simulink model "MAIN_IC_TEST_original"  (R2020b)
settings: Solver=ode4  StartTime=0.0  StopTime=inf  FixedStep=1/1000  RelTol=1e-3
libraries: speedgoatlib_IO691 x12, canmsglib x10, simulink x2
(part 2 of 2)

== matlab function MAIN_IC_TEST_original/to_dPolar1 ==
  data: theta1 input; theta2 input; dr output; dphi output; dtheta1 input; dtheta2 input
function [dr,dphi] = Velocity(theta1,theta2,dtheta1,dtheta2)
%VELOCITY
%    [DR,DPHI] = VELOCITY(THETA1,THETA2,DTHETA1,DTHETA2)

%    This function was generated by the Symbolic Math Toolbox version 8.6.
%    13-May-2022 14:39:46

dr = dtheta1.*1.0./sqrt((sin(acos(sqrt((sin(theta1-pi./2.0).*(3.7e+1./2.0e+2)+sin(theta2+pi./2.0).*(3.7e+1./2.0e+2)).^2+abs(cos(theta1-pi./2.0).*(3.7e+1./2.0e+2)+cos(theta2+pi./2.0).*(3.7e+1./2.0e+2)+3.0./2.5e+1).^2).*(5.0e+1./3.7e+1))+atan2(sin(theta1-pi./2.0).*(-3.7e+1./2.0e+2)-sin(theta2+pi./2.0).*(3.7e+1./2.0e+2),abs(cos(theta1-pi./2.0).*(3.7e+1./2.0e+2)+cos(theta2+pi./2.0).*(3.7e+1./2.0e+2)+3.0./2.5e+1))+7.170057008954915e-2).*4.187654330625071e-1+sin(theta2+pi./2.0).*(3.7e+1./2.0e+2)).^2+(cos(acos(sqrt((sin(theta1-pi./2.0).*(3.7e+1./2.0e+2)+sin(theta2+pi./2.0).*(3.7e+1./2.0e+2)).^2+abs(cos(theta1-pi./2.0).*(3.7e+1./2.0e+2)+cos(theta2+pi./2.0).*(3.7e+1./2.0e+2)+3.0./2.5e+1).^2).*(5.0e+1./3.7e+1))+atan2(sin(theta1-pi./2.0).*(-3.7e+1./2.0e+2)-sin(theta2+pi./2.0).*(3.7e+1./2.0e+2),abs(cos(theta1-pi./2.0).*(3.7e+1./2.0e+2)+cos(theta2+pi./2.0).*(3.7e+1./2.0e+2)+3.0./2.5e+1))+7.170057008954915e-2).*(-4.187654330625071e-1)+cos(theta2+pi./2.0).*(3.7e+1./2.0e+2)+3.0./5.0e+1).^2).*(sin(acos(sqrt((sin(theta1-pi./2.0).*(3.7e+1./2.0e+2)+sin(theta2+pi./2.0).*(3.7e+1./2.0e+2)).^2+abs(cos(theta1-pi./2.0).*(3.7e+1./2.0e+2)+cos(theta2+pi./2.0).*(3.7e+1./2.0e+2)+3.0./2.5e+1).^2).*(5.0e+1./3.7e+1))+atan2(sin(theta1-pi./2.0).*(-3.7e+1./2.0e+2)-sin(theta2+pi./2.0).*(3.7e+1./2.0e+2),abs(cos(theta1-pi./2.0).*(3.7e+1./2.0e+2)+cos(theta2+pi./2.0).*(3.7e+1./2.0e+2)+3.0./2.5e+1))+7.170057008954915e-2).*(1.0./sqrt((sin(theta1-pi./2.0).*(3.7e+1./2.0e+2)+sin(theta2+pi./2.0).*(3.7e+1./2.0e+2)).^2+abs(cos(theta1-pi./2.0).*(3.7e+1./2.0e+2)+cos(theta2+pi./2.0).*(3.7e+1./2.0e+2)+3.0./2.5e+1).^2).*(cos(theta1-pi./2.0).*(sin(theta1-pi./2.0).*(3.7e+1./2.0e+2)+sin(theta2+pi./2.0).*(3.7e+1./2.0e+2)).*(3.7e+1./1.0e+2)-abs(cos(theta1-pi./2.0).*(3.7e+1./2.0e+2)+cos(theta2+pi./2.0).*(3.7e+1./2.0e+2)+3.0./2.5e+1).*sign(cos(theta1-pi./2.0).*(3.7e+1./2.0e+2)+cos(theta2+pi./2.0).*(3.7e+1./2.0e+2)+3.0./2.5e+1).*sin(theta1-pi./2.0).*(3.7e+1./1.0e+2)).*1.0./sqrt((sin(theta1-pi./2.0).*(3.7e+1./2.0e+2)+sin(theta2+pi./2.0).*(3.7e+1./2.0e+2)).^2.*(-1.826150474799123)-abs(cos(theta1-pi./2.0).*(3.7e+1./2.0e+2)+cos(theta2+pi./2.0).*(3.7e+1./2.0e+2)+3.0./2.5e+1).^2.*1.826150474799123+1.0).*(2.5e+1./3.7e+1)+(abs(cos(theta1-pi./2.0).*(3.7e+1./2.0e+2)+cos(theta2+pi./2.0).*(3.7e+1./2.0e+2)+3.0./2.5e+1).^2.*((cos(theta1-pi./2.0).*(3.7e+1./2.0e+2))./abs(cos(theta1-pi./2.0).*(3.7e+1./2.0e+2)+cos(theta2+pi./2.0).*(3.7e+1./2.0e+2)+3.0./2.5e+1)+1.0./abs(cos(theta1-pi./2.0).*(3.7e+1./2.0e+2)+cos(theta2+pi./2.0).*(3.7e+1./2.0e+2)+3.0./2.5e+1).^2.*sign(cos(theta1-pi./2.0).*(3.7e+1./2.0e+2)+cos(theta2+pi./2.0).*(3.7e+1./2.0e+2)+3.0./2.5e+1).*sin(theta1-pi./2.0).*(sin(theta1-pi./2.0).*(3.7e+1./2.0e+2)+sin(theta2+pi./2.0).*(3.7e+1./2.0e+2)).*(3.7e+1./2.0e+2)))./((sin(theta1-pi./2.0).*(3.7e+1./2.0e+2)+sin(theta2+pi./2.0).*(3.7e+1./2.0e+2)).^2+abs(cos(theta1-pi./2.0).*(3.7e+1./2.0e+2)+cos(theta2+pi./2.0).*(3.7e+1./2.0e+2)+3.0./2.5e+1).^2)).*(cos(acos(sqrt((sin(theta1-pi./2.0).*(3.7e+1./2.0e+2)+sin(theta2+pi./2.0).*(3.7e+1./2.0e+2)).^2+abs(cos(theta1-pi./2.0).*(3.7e+1./2.0e+2)+cos(theta2+pi./2.0).*(3.7e+1./2.0e+2)+3.0./2.5e+1).^2).*(5.0e+1./3.7e+1))+atan2(sin(theta1-pi./2.0).*(-3.7e+1./2.0e+2)-sin(theta2+pi./2.0).*(3.7e+1./2.0e+2),abs(cos(theta1-pi./2.0).*(3.7e+1./2.0e+2)+cos(theta2+pi./2.0).*(3.7e+1./2.0e+2)+3.0./2.5e+1))+7.170057008954915e-2).*(-4.187654330625071e-1)+cos(theta2+pi./2.0).*(3.7e+1./2.0e+2)+3.0./5.0e+1).*8.375308661250142e-1+cos(acos(sqrt((sin(theta1-pi./2.0).*(3.7e+1./2.0e+2)+sin(theta2+pi./2.0).*(3.7e+1./2.0e+2)).^2+abs(cos(theta1-pi./2.0).*(3.7e+1./2.0e+2)+cos(theta2+pi./2.0).*(3.7e+1./2.0e+2)+3.0./2.5e+1).^2).*(5.0e+1./3.7e+1))+atan2(sin(theta1-pi./2.0).*(-3.7e+1./2.0e+2)-sin(theta2+pi./2.0).*(3.7e+1./2.0e+2),abs(cos(theta1-pi./2.0).*(3.7e+1./2.0e+2)+cos(theta2+pi./2.0).*(3.7e+1./2.0e+2)+3.0./2.5e+1))+7.170057008954915e-2).*(1.0./sqrt((sin(theta1-pi./2.0).*(3.7e+1./2.0e+2)+sin(theta2+pi./2.0).*(3.7e+1./2.0e+2)).^2+abs(cos(theta1-pi./2.0).*(3.7e+1./2.0e+2)+cos(theta2+pi./2.0).*(3.7e+1./2.0e+2)+3.0./2.5e+1).^2).*(cos(theta1-pi./2.0).*(sin(theta1-pi./2.0).*(3.7e+1./2.0e+2)+sin(theta2+pi./2.0).*(3.7e+1./2.0e+2)).*(3.7e+1./1.0e+2)-abs(cos(theta1-pi./2.0).*(3.7e+1./2.0e+2)+cos(theta2+pi./2.0).*(3.7e+1./2.0e+2)+3.0./2.5e+1).*sign(cos(theta1-pi./2.0).*(3.7e+1./2.0e+2)+cos(theta2+pi./2.0).*(3.7e+1./2.0e+2)+3.0./2.5e+1).*sin(theta1-pi./2.0).*(3.7e+1./1.0e+2)).*1.0./sqrt((sin(theta1-pi./2.0).*(3.7e+1./2.0e+2)+sin(theta2+pi./2.0).*(3.7e+1./2.0e+2)).^2.*(-1.826150474799123)-abs(cos(theta1-pi./2.0).*(3.7e+1./2.0e+2)+cos(theta2+pi./2.0).*(3.7e+1./2.0e+2)+3.0./2.5e+1).^2.*1.826150474799123+1.0).*(2.5e+1./3.7e+1)+(abs(cos(theta1-pi./2.0).*(3.7e+1./2.0e+2)+cos(theta2+pi./2.0).*(3.7e+1./2.0e+2)+3.0./2.5e+1).^2.*((cos(theta1-pi./2.0).*(3.7e+1./2.0e+2))./abs(cos(theta1-pi./2.0).*(3.7e+1./2.0e+2)+cos(theta2+pi./2.0).*(3.7e+1./2.0e+2)+3.0./2.5e+1)+1.0./abs(cos(theta1-pi./2.0).*(3.7e+1./2.0e+2)+cos(theta2+pi./2.0).*(3.7e+1./2.0e+2)+3.0./2.5e+1).^2.*sign(cos(theta1-pi./2.0).*(3.7e+1./2.0e+2)+cos(theta2+pi./2.0).*(3.7e+1./2.0e+2)+3.0./2.5e+1).*sin(theta1-pi./2.0).*(sin(theta1-pi./2.0).*(3.7e+1./2.0e+2)+sin(theta2+pi./2.0).*(3.7e+1./2.0e+2)).*(3.7e+1./2.0e+2)))./((sin(theta1-pi./2.0).*(3.7e+1./2.0e+2)+sin(theta2+pi./2.0).*(3.7e+1./2.0e+2)).^2+abs(cos(theta1-pi./2.0).*(3.7e+1./2.0e+2)+cos(theta2+pi./2.0).*(3.7e+1./2.0e+2)+3.0./2.5e+1).^2)).*(sin(acos(sqrt((sin(theta1-pi./2.0).*(3.7e+1./2.0e+2)+sin(theta2+pi./2.0).*(3.7e+1./2.0e+2)).^2+abs(cos(theta1-pi./2.0).*(3.7e+1./2.0e+2)+cos(theta2+pi./2.0).*(3.7e+1./2.0e+2)+3.0./2.5e+1).^2).*(5.0e+1./3.7e+1))+atan2(sin(theta1-pi./2.0).*(-3.7e+1./2.0e+2)-sin(theta2+pi./2.0).*(3.7e+1./2.0e+2),abs(cos(theta1-pi./2.0).*(3.7e+1./2.0e+2)+cos(theta2+pi./2.0).*(3.7e+1./2.0e+2)+3.0./2.5e+1))+7.170057008954915e-2).*4.187654330625071e-1+sin(theta2+pi./2.0).*(3.7e+1./2.0e+2)).*8.375308661250142e-1).*(-1.0./2.0)+(dtheta2.*1.0./sqrt((sin(acos(sqrt((sin(theta1-pi./2.0).*(3.7e+1./2.0e+2)+sin(theta2+pi./2.0).*(3.7e+1./2.0e+2)).^2+abs(cos(theta1-pi./2.0).*(3.7e+1./2.0e+2)+cos(theta2+pi./2.0).*(3.7e+1./2.0e+2)+3.0./2.5e+1).^2).*(5.0e+1./3.7e+1))+atan2(sin(theta1-pi./2.0).*(-3.7e+1./2.0e+2)-sin(theta2+pi./2.0).*(3.7e+1./2.0e+2),abs(cos(theta1-pi./2.0).*(3.7e+1./2.0e+2)+cos(theta2+pi./2.0).*(3.7e+1./2.0e+2)+3.0./2.5e+1))+7.170057008954915e-2).*4.187654330625071e-1+sin(theta2+pi./2.0).*(3.7e+1./2.0e+2)).^2+(cos(acos(sqrt((sin(theta1-pi./2.0).*(3.7e+1./2.0e+2)+sin(theta2+pi./2.0).*(3.7e+1./2.0e+2)).^2+abs(cos(theta1-pi./2.0).*(3.7e+1./2.0e+2)+cos(theta2+pi./2.0).*(3.7e+1./2.0e+2)+3.0./2.5e+1).^2).*(5.0e+1./3.7e+1))+atan2(sin(theta1-pi./2.0).*(-3.7e+1./2.0e+2)-sin(theta2+pi./2.0).*(3.7e+1./2.0e+2),abs(cos(theta1-pi./2.0).*(3.7e+1./2.0e+2)+cos(theta2+pi./2.0).*(3.7e+1./2.0e+2)+3.0./2.5e+1))+7.170057008954915e-2).*(-4.187654330625071e-1)+cos(theta2+pi./2.0).*(3.7e+1./2.0e+2)+3.0./5.0e+1).^2).*((cos(theta2+pi./2.0).*(3.7e+1./2.0e+2)-cos(acos(sqrt((sin(theta1-pi./2.0).*(3.7e+1./2.0e+2)+sin(theta2+pi./2.0).*(3.7e+1./2.0e+2)).^2+abs(cos(theta1-pi./2.0).*(3.7e+1./2.0e+2)+cos(theta2+pi./2.0).*(3.7e+1./2.0e+2)+3.0./2.5e+1).^2).*(5.0e+1./3.7e+1))+atan2(sin(theta1-pi./2.0).*(-3.7e+1./2.0e+2)-sin(theta2+pi./2.0).*(3.7e+1./2.0e+2),abs(cos(theta1-pi./2.0).*(3.7e+1./2.0e+2)+cos(theta2+pi./2.0).*(3.7e+1./2.0e+2)+3.0./2.5e+1))+7.170057008954915e-2).*(1.0./sqrt((sin(theta1-pi./2.0).*(3.7e+1./2.0e+2)+sin(theta2+pi./2.0).*(3.7e+1./2.0e+2)).^2+abs(cos(theta1-pi./2.0).*(3.7e+1./2.0e+2)+cos(theta2+pi./2.0).*(3.7e+1./2.0e+2)+3.0./2.5e+1).^2).*(cos(theta2+pi./2.0).*(sin(theta1-pi./2.0).*(3.7e+1./2.0e+2)+sin(theta2+pi./2.0).*(3.7e+1./2.0e+2)).*(3.7e+1./1.0e+2)-abs(cos(theta1-pi./2.0).*(3.7e+1./2.0e+2)+cos(theta2+pi./2.0).*(3.7e+1./2.0e+2)+3.0./2.5e+1).*sign(cos(theta1-pi./2.0).*(3.7e+1./2.0e+2)+cos(theta2+pi./2.0).*(3.7e+1./2.0e+2)+3.0./2.5e+1).*sin(theta2+pi./2.0).*(3.7e+1./1.0e+2)).*1.0./sqrt((sin(theta1-pi./2.0).*(3.7e+1./2.0e+2)+sin(theta2+pi./2.0).*(3.7e+1./2.0e+2)).^2.*(-1.826150474799123)-abs(cos(theta1-pi./2.0).*(3.7e+1./2.0e+2)+cos(theta2+pi./2.0).*(3.7e+1./2.0e+2)+3.0./2.5e+1).^2.*1.826150474799123+1.0).*(2.5e+1./3.7e+1)+(abs(cos(theta1-pi./2.0).*(3.7e+1./2.0e+2)+cos(theta2+pi./2.0).*(3.7e+1./2.0e+2)+3.0./2.5e+1).^2.*((cos(theta2+pi./2.0).*(3.7e+1./2.0e+2))./abs(cos(theta1-pi./2.0).*(3.7e+1./2.0e+2)+cos(theta2+pi./2.0).*(3.7e+1./2.0e+2)+3.0./2.5e+1)+1.0./abs(cos(theta1-pi./2.0).*(3.7e+1./2.0e+2)+cos(theta2+pi./2.0).*(3.7e+1./2.0e+2)+3.0./2.5e+1).^2.*sign(cos(theta1-pi./2.0).*(3.7e+1./2.0e+2)+cos(theta2+pi./2.0).*(3.7e+1./2.0e+2)+3.0./2.5e+1).*sin(theta2+pi./2.0).*(sin(theta1-pi./2.0).*(3.7e+1./2.0e+2)+sin(theta2+pi./2.0).*(3.7e+1./2.0e+2)).*(3.7e+1./2.0e+2)))./((sin(theta1-pi./2.0).*(3.7e+1./2.0e+2)+sin(theta2+pi./2.0).*(3.7e+1./2.0e+2)).^2+abs(cos(theta1-pi./2.0).*(3.7e+1./2.0e+2)+cos(theta2+pi./2.0).*(3.7e+1./2.0e+2)+3.0./2.5e+1).^2)).*4.187654330625071e-1).*(sin(acos(sqrt((sin(theta1-pi./2.0).*(3.7e+1./2.0e+2)+sin(theta2+pi./2.0).*(3.7e+1./2.0e+2)).^2+abs(cos(theta1-pi./2.0).*(3.7e+1./2.0e+2)+cos(theta2+pi./2.0).*(3.7e+1./2.0e+2)+3.0./2.5e+1).^2).*(5.0e+1./3.7e+1))+atan2(sin(theta1-pi./2.0).*(-3.7e+1./2.0e+2)-sin(theta2+pi./2.0).*(3.7e+1./2.0e+2),abs(cos(theta1-pi./2.0).*(3.7e+1./2.0e+2)+cos(theta2+pi./2.0).*(3.7e+1./2.0e+2)+3.0./2.5e+1))+7.170057008954915e-2).*4.187654330625071e-1+sin(theta2+pi./2.0).*(3.7e+1./2.0e+2)).*2.0-(sin(theta2+pi./2.0).*(3.7e+1./2.0e+2)+sin(acos(sqrt((sin(theta1-pi./2.0).*(3.7e+1./2.0e+2)+sin(theta2+pi./2.0).*(3.7e+1./2.0e+2)).^2+abs(cos(theta1-pi./2.0).*(3.7e+1./2.0e+2)+cos(theta2+pi./2.0).*(3.7e+1./2.0e+2)+3.0./2.5e+1).^2).*(5.0e+1./3.7e+1))+atan2(sin(theta1-pi./2.0).*(-3.7e+1./2.0e+2)-sin(theta2+pi./2.0).*(3.7e+1./2.0e+2),abs(cos(theta1-pi./2.0).*(3.7e+1./2.0e+2)+cos(theta2+pi./2.0).*(3.7e+1./2.0e+2)+3.0./2.5e+1))+7.170057008954915e-2).*(1.0./sqrt((sin(theta1-pi./2.0).*(3.7e+1./2.0e+2)+sin(theta2+pi./2.0).*(3.7e+1./2.0e+2)).^2+abs(cos(theta1-pi./2.0).*(3.7e+1./2.0e+2)+cos(theta2+pi./2.0).*(3.7e+1./2.0e+2)+3.0./2.5e+1).^2).*(cos(theta2+pi./2.0).*(sin(theta1-pi./2.0).*(3.7e+1./2.0e+2)+sin(theta2+pi./2.0).*(3.7e+1./2.0e+2)).*(3.7e+1./1.0e+2)-abs(cos(theta1-pi./2.0).*(3.7e+1./2.0e+2)+cos(theta2+pi./2.0).*(3.7e+1./2.0e+2)+3.0./2.5e+1).*sign(cos(theta1-pi./2.0).*(3.7e+1./2.0e+2)+cos(theta2+pi./2.0).*(3.7e+1./2.0e+2)+3.0./2.5e+1).*sin(theta2+pi./2.0).*(3.7e+1./1.0e+2)).*1.0./sqrt((sin(theta1-pi./2.0).*(3.7e+1./2.0e+2)+sin(theta2+pi./2.0).*(3.7e+1./2.0e+2)).^2.*(-1.826150474799123)-abs(cos(theta1-pi./2.0).*(3.7e+1./2.0e+2)+cos(theta2+pi./2.0).*(3.7e+1./2.0e+2)+3.0./2.5e+1).^2.*1.826150474799123+1.0).*(2.5e+1./3.7e+1)+(abs(cos(theta1-pi./2.0).*(3.7e+1./2.0e+2)+cos(theta2+pi./2.0).*(3.7e+1./2.0e+2)+3.0./2.5e+1).^2.*((cos(theta2+pi./2.0).*(3.7e+1./2.0e+2))./abs(cos(theta1-pi./2.0).*(3.7e+1./2.0e+2)+cos(theta2+pi./2.0).*(3.7e+1./2.0e+2)+3.0./2.5e+1)+1.0./abs(cos(theta1-pi./2.0).*(3.7e+1./2.0e+2)+cos(theta2+pi./2.0).*(3.7e+1./2.0e+2)+3.0./2.5e+1).^2.*sign(cos(theta1-pi./2.0).*(3.7e+1./2.0e+2)+cos(theta2+pi./2.0).*(3.7e+1./2.0e+2)+3.0./2.5e+1).*sin(theta2+pi./2.0).*(sin(theta1-pi./2.0).*(3.7e+1./2.0e+2)+sin(theta2+pi./2.0).*(3.7e+1./2.0e+2)).*(3.7e+1./2.0e+2)))./((sin(theta1-pi./2.0).*(3.7e+1./2.0e+2)+sin(theta2+pi./2.0).*(3.7e+1./2.0e+2)).^2+abs(cos(theta1-pi./2.0).*(3.7e+1./2.0e+2)+cos(theta2+pi./2.0).*(3.7e+1./2.0e+2)+3.0./2.5e+1).^2)).*4.187654330625071e-1).*(cos(acos(sqrt((sin(theta1-pi./2.0).*(3.7e+1./2.0e+2)+sin(theta2+pi./2.0).*(3.7e+1./2.0e+2)).^2+abs(cos(theta1-pi./2.0).*(3.7e+1./2.0e+2)+cos(theta2+pi./2.0).*(3.7e+1./2.0e+2)+3.0./2.5e+1).^2).*(5.0e+1./3.7e+1))+atan2(sin(theta1-pi./2.0).*(-3.7e+1./2.0e+2)-sin(theta2+pi./2.0).*(3.7e+1./2.0e+2),abs(cos(theta1-pi./2.0).*(3.7e+1./2.0e+2)+cos(theta2+pi./2.0).*(3.7e+1./2.0e+2)+3.0./2.5e+1))+7.170057008954915e-2).*(-4.187654330625071e-1)+cos(theta2+pi./2.0).*(3.7e+1./2.0e+2)+3.0./5.0e+1).*2.0))./2.0;
if nargout > 1
    dphi = (dtheta1.*((cos(acos(sqrt((sin(theta1-pi./2.0).*(3.7e+1./2.0e+2)+sin(theta2+pi./2.0).*(3.7e+1./2.0e+2)).^2+abs(cos(theta1-pi./2.0).*(3.7e+1./2.0e+2)+cos(theta2+pi./2.0).*(3.7e+1./2.0e+2)+3.0./2.5e+1).^2).*(5.0e+1./3.7e+1))+atan2(sin(theta1-pi./2.0).*(-3.7e+1./2.0e+2)-sin(theta2+pi./2.0).*(3.7e+1./2.0e+2),abs(cos(theta1-pi./2.0).*(3.7e+1./2.0e+2)+cos(theta2+pi./2.0).*(3.7e+1./2.0e+2)+3.0./2.5e+1))+7.170057008954915e-2).*(1.0./sqrt((sin(theta1-pi./2.0).*(3.7e+1./2.0e+2)+sin(theta2+pi./2.0).*(3.7e+1./2.0e+2)).^2+abs(cos(theta1-pi./2.0).*(3.7e+1./2.0e+2)+cos(theta2+pi./2.0).*(3.7e+1./2.0e+2)+3.0./2.5e+1).^2).*(cos(theta1-pi./2.0).*(sin(theta1-pi./2.0).*(3.7e+1./2.0e+2)+sin(theta2+pi./2.0).*(3.7e+1./2.0e+2)).*(3.7e+1./1.0e+2)-abs(cos(theta1-pi./2.0).*(3.7e+1./2.0e+2)+cos(theta2+pi./2.0).*(3.7e+1./2.0e+2)+3.0./2.5e+1).*sign(cos(theta1-pi./2.0).*(3.7e+1./2.0e+2)+cos(theta2+pi./2.0).*(3.7e+1./2.0e+2)+3.0./2.5e+1).*sin(theta1-pi./2.0).*(3.7e+1./1.0e+2)).*1.0./sqrt((sin(theta1-pi./2.0).*(3.7e+1./2.0e+2)+sin(theta2+pi./2.0).*(3.7e+1./2.0e+2)).^2.*(-1.826150474799123)-abs(cos(theta1-pi./2.0).*(3.7e+1./2.0e+2)+cos(theta2+pi./2.0).*(3.7e+1./2.0e+2)+3.0./2.5e+1).^2.*1.826150474799123+1.0).*(2.5e+1./3.7e+1)+(abs(cos(theta1-pi./2.0).*(3.7e+1./2.0e+2)+cos(theta2+pi./2.0).*(3.7e+1./2.0e+2)+3.0./2.5e+1).^2.*((cos(theta1-pi./2.0).*(3.7e+1./2.0e+2))./abs(cos(theta1-pi./2.0).*(3.7e+1./2.0e+2)+cos(theta2+pi./2.0).*(3.7e+1./2.0e+2)+3.0./2.5e+1)+1.0./abs(cos(theta1-pi./2.0).*(3.7e+1./2.0e+2)+cos(theta2+pi./2.0).*(3.7e+1./2.0e+2)+3.0./2.5e+1).^2.*sign(cos(theta1-pi./2.0).*(3.7e+1./2.0e+2)+cos(theta2+pi./2.0).*(3.7e+1./2.0e+2)+3.0./2.5e+1).*sin(theta1-pi./2.0).*(sin(theta1-pi./2.0).*(3.7e+1./2.0e+2)+sin(theta2+pi./2.0).*(3.7e+1./2.0e+2)).*(3.7e+1./2.0e+2)))./((sin(theta1-pi./2.0).*(3.7e+1./2.0e+2)+sin(theta2+pi./2.0).*(3.7e+1./2.0e+2)).^2+abs(cos(theta1-pi./2.0).*(3.7e+1./2.0e+2)+cos(theta2+pi./2.0).*(3.7e+1./2.0e+2)+3.0./2.5e+1).^2)).*4.187654330625071e-1)./(cos(acos(sqrt((sin(theta1-pi./2.0).*(3.7e+1./2.0e+2)+sin(theta2+pi./2.0).*(3.7e+1./2.0e+2)).^2+abs(cos(theta1-pi./2.0).*(3.7e+1./2.0e+2)+cos(theta2+pi./2.0).*(3.7e+1./2.0e+2)+3.0./2.5e+1).^2).*(5.0e+1./3.7e+1))+atan2(sin(theta1-pi./2.0).*(-3.7e+1./2.0e+2)-sin(theta2+pi./2.0).*(3.7e+1./2.0e+2),abs(cos(theta1-pi./2.0).*(3.7e+1./2.0e+2)+cos(theta2+pi./2.0).*(3.7e+1./2.0e+2)+3.0./2.5e+1))+7.170057008954915e-2).*(-4.187654330625071e-1)+cos(theta2+pi./2.0).*(3.7e+1./2.0e+2)+3.0./5.0e+1)-sin(acos(sqrt((sin(theta1-pi./2.0).*(3.7e+1./2.0e+2)+sin(theta2+pi./2.0).*(3.7e+1./2.0e+2)).^2+abs(cos(theta1-pi./2.0).*(3.7e+1./2.0e+2)+cos(theta2+pi./2.0).*(3.7e+1./2.0e+2)+3.0./2.5e+1).^2).*(5.0e+1./3.7e+1))+atan2(sin(theta1-pi./2.0).*(-3.7e+1./2.0e+2)-sin(theta2+pi./2.0).*(3.7e+1./2.0e+2),abs(cos(theta1-pi./2.0).*(3.7e+1./2.0e+2)+cos(theta2+pi./2.0).*(3.7e+1./2.0e+2)+3.0./2.5e+1))+7.170057008954915e-2).*(1.0./sqrt((sin(theta1-pi./2.0).*(3.7e+1./2.0e+2)+sin(theta2+pi./2.0).*(3.7e+1./2.0e+2)).^2+abs(cos(theta1-pi./2.0).*(3.7e+1./2.0e+2)+cos(theta2+pi./2.0).*(3.7e+1./2.0e+2)+3.0./2.5e+1).^2).*(cos(theta1-pi./2.0).*(sin(theta1-pi./2.0).*(3.7e+1./2.0e+2)+sin(theta2+pi./2.0).*(3.7e+1./2.0e+2)).*(3.7e+1./1.0e+2)-abs(cos(theta1-pi./2.0).*(3.7e+1./2.0e+2)+cos(theta2+pi./2.0).*(3.7e+1./2.0e+2)+3.0./2.5e+1).*sign(cos(theta1-pi./2.0).*(3.7e+1./2.0e+2)+cos(theta2+pi./2.0).*(3.7e+1./2.0e+2)+3.0./2.5e+1).*sin(theta1-pi./2.0).*(3.7e+1./1.0e+2)).*1.0./sqrt((sin(theta1-pi./2.0).*(3.7e+1./2.0e+2)+sin(theta2+pi./2.0).*(3.7e+1./2.0e+2)).^2.*(-1.826150474799123)-abs(cos(theta1-pi./2.0).*(3.7e+1./2.0e+2)+cos(theta2+pi./2.0).*(3.7e+1./2.0e+2)+3.0./2.5e+1).^2.*1.826150474799123+1.0).*(2.5e+1./3.7e+1)+(abs(cos(theta1-pi./2.0).*(3.7e+1./2.0e+2)+cos(theta2+pi./2.0).*(3.7e+1./2.0e+2)+3.0./2.5e+1).^2.*((cos(theta1-pi./2.0).*(3.7e+1./2.0e+2))./abs(cos(theta1-pi./2.0).*(3.7e+1./2.0e+2)+cos(theta2+pi./2.0).*(3.7e+1./2.0e+2)+3.0./2.5e+1)+1.0./abs(cos(theta1-pi./2.0).*(3.7e+1./2.0e+2)+cos(theta2+pi./2.0).*(3.7e+1./2.0e+2)+3.0./2.5e+1).^2.*sign(cos(theta1-pi./2.0).*(3.7e+1./2.0e+2)+cos(theta2+pi./2.0).*(3.7e+1./2.0e+2)+3.0./2.5e+1).*sin(theta1-pi./2.0).*(sin(theta1-pi./2.0).*(3.7e+1./2.0e+2)+sin(theta2+pi./2.0).*(3.7e+1./2.0e+2)).*(3.7e+1./2.0e+2)))./((sin(theta1-pi./2.0).*(3.7e+1./2.0e+2)+sin(theta2+pi./2.0).*(3.7e+1./2.0e+2)).^2+abs(cos(theta1-pi./2.0).*(3.7e+1./2.0e+2)+cos(theta2+pi./2.0).*(3.7e+1./2.0e+2)+3.0./2.5e+1).^2)).*(sin(acos(sqrt((sin(theta1-pi./2.0).*(3.7e+1./2.0e+2)+sin(theta2+pi./2.0).*(3.7e+1./2.0e+2)).^2+abs(cos(theta1-pi./2.0).*(3.7e+1./2.0e+2)+cos(theta2+pi./2.0).*(3.7e+1./2.0e+2)+3.0./2.5e+1).^2).*(5.0e+1./3.7e+1))+atan2(sin(theta1-pi./2.0).*(-3.7e+1./2.0e+2)-sin(theta2+pi./2.0).*(3.7e+1./2.0e+2),abs(cos(theta1-pi./2.0).*(3.7e+1./2.0e+2)+cos(theta2+pi./2.0).*(3.7e+1./2.0e+2)+3.0./2.5e+1))+7.170057008954915e-2).*4.187654330625071e-1+sin(theta2+pi./2.0).*(3.7e+1./2.0e+2)).*1.0./(cos(acos(sqrt((sin(theta1-pi./2.0).*(3.7e+1./2.0e+2)+sin(theta2+pi./2.0).*(3.7e+1./2.0e+2)).^2+abs(cos(theta1-pi./2.0).*(3.7e+1./2.0e+2)+cos(theta2+pi./2.0).*(3.7e+1./2.0e+2)+3.0./2.5e+1).^2).*(5.0e+1./3.7e+1))+atan2(sin(theta1-pi./2.0).*(-3.7e+1./2.0e+2)-sin(theta2+pi./2.0).*(3.7e+1./2.0e+2),abs(cos(theta1-pi./2.0).*(3.7e+1./2.0e+2)+cos(theta2+pi./2.0).*(3.7e+1./2.0e+2)+3.0./2.5e+1))+7.170057008954915e-2).*(-4.187654330625071e-1)+cos(theta2+pi./2.0).*(3.7e+1./2.0e+2)+3.0./5.0e+1).^2.*4.187654330625071e-1).*(cos(acos(sqrt((sin(theta1-pi./2.0).*(3.7e+1./2.0e+2)+sin(theta2+pi./2.0).*(3.7e+1./2.0e+2)).^2+abs(cos(theta1-pi./2.0).*(3.7e+1./2.0e+2)+cos(theta2+pi./2.0).*(3.7e+1./2.0e+2)+3.0./2.5e+1).^2).*(5.0e+1./3.7e+1))+atan2(sin(theta1-pi./2.0).*(-3.7e+1./2.0e+2)-sin(theta2+pi./2.0).*(3.7e+1./2.0e+2),abs(cos(theta1-pi./2.0).*(3.7e+1./2.0e+2)+cos(theta2+pi./2.0).*(3.7e+1./2.0e+2)+3.0./2.5e+1))+7.170057008954915e-2).*(-4.187654330625071e-1)+cos(theta2+pi./2.0).*(3.7e+1./2.0e+2)+3.0./5.0e+1).^2)./((sin(acos(sqrt((sin(theta1-pi./2.0).*(3.7e+1./2.0e+2)+sin(theta2+pi./2.0).*(3.7e+1./2.0e+2)).^2+abs(cos(theta1-pi./2.0).*(3.7e+1./2.0e+2)+cos(theta2+pi./2.0).*(3.7e+1./2.0e+2)+3.0./2.5e+1).^2).*(5.0e+1./3.7e+1))+atan2(sin(theta1-pi./2.0).*(-3.7e+1./2.0e+2)-sin(theta2+pi./2.0).*(3.7e+1./2.0e+2),abs(cos(theta1-pi./2.0).*(3.7e+1./2.0e+2)+cos(theta2+pi./2.0).*(3.7e+1./2.0e+2)+3.0./2.5e+1))+7.170057008954915e-2).*4.187654330625071e-1+sin(theta2+pi./2.0).*(3.7e+1./2.0e+2)).^2+(cos(acos(sqrt((sin(theta1-pi./2.0).*(3.7e+1./2.0e+2)+sin(theta2+pi./2.0).*(3.7e+1./2.0e+2)).^2+abs(cos(theta1-pi./2.0).*(3.7e+1./2.0e+2)+cos(theta2+pi./2.0).*(3.7e+1./2.0e+2)+3.0./2.5e+1).^2).*(5.0e+1./3.7e+1))+atan2(sin(theta1-pi./2.0).*(-3.7e+1./2.0e+2)-sin(theta2+pi./2.0).*(3.7e+1./2.0e+2),abs(cos(theta1-pi./2.0).*(3.7e+1./2.0e+2)+cos(theta2+pi./2.0).*(3.7e+1./2.0e+2)+3.0./2.5e+1))+7.170057008954915e-2).*(-4.187654330625071e-1)+cos(theta2+pi./2.0).*(3.7e+1./2.0e+2)+3.0./5.0e+1).^2)-(dtheta2.*((cos(theta2+pi./2.0).*(3.7e+1./2.0e+2)-cos(acos(sqrt((sin(theta1-pi./2.0).*(3.7e+1./2.0e+2)+sin(theta2+pi./2.0).*(3.7e+1./2.0e+2)).^2+abs(cos(theta1-pi./2.0).*(3.7e+1./2.0e+2)+cos(theta2+pi./2.0).*(3.7e+1./2.0e+2)+3.0./2.5e+1).^2).*(5.0e+1./3.7e+1))+atan2(sin(theta1-pi./2.0).*(-3.7e+1./2.0e+2)-sin(theta2+pi./2.0).*(3.7e+1./2.0e+2),abs(cos(theta1-pi./2.0).*(3.7e+1./2.0e+2)+cos(theta2+pi./2.0).*(3.7e+1./2.0e+2)+3.0./2.5e+1))+7.170057008954915e-2).*(1.0./sqrt((sin(theta1-pi./2.0).*(3.7e+1./2.0e+2)+sin(theta2+pi./2.0).*(3.7e+1./2.0e+2)).^2+abs(cos(theta1-pi./2.0).*(3.7e+1./2.0e+2)+cos(theta2+pi./2.0).*(3.7e+1./2.0e+2)+3.0./2.5e+1).^2).*(cos(theta2+pi./2.0).*(sin(theta1-pi./2.0).*(3.7e+1./2.0e+2)+sin(theta2+pi./2.0).*(3.7e+1./2.0e+2)).*(3.7e+1./1.0e+2)-abs(cos(theta1-pi./2.0).*(3.7e+1./2.0e+2)+cos(theta2+pi./2.0).*(3.7e+1./2.0e+2)+3.0./2.5e+1).*sign(cos(theta1-pi./2.0).*(3.7e+1./2.0e+2)+cos(theta2+pi./2.0).*(3.7e+1./2.0e+2)+3.0./2.5e+1).*sin(theta2+pi./2.0).*(3.7e+1./1.0e+2)).*1.0./sqrt((sin(theta1-pi./2.0).*(3.7e+1./2.0e+2)+sin(theta2+pi./2.0).*(3.7e+1./2.0e+2)).^2.*(-1.826150474799123)-abs(cos(theta1-pi./2.0).*(3.7e+1./2.0e+2)+cos(theta2+pi./2.0).*(3.7e+1./2.0e+2)+3.0./2.5e+1).^2.*1.826150474799123+1.0).*(2.5e+1./3.7e+1)+(abs(cos(theta1-pi./2.0).*(3.7e+1./2.0e+2)+cos(theta2+pi./2.0).*(3.7e+1./2.0e+2)+3.0./2.5e+1).^2.*((cos(theta2+pi./2.0).*(3.7e+1./2.0e+2))./abs(cos(theta1-pi./2.0).*(3.7e+1./2.0e+2)+cos(theta2+pi./2.0).*(3.7e+1./2.0e+2)+3.0./2.5e+1)+1.0./abs(cos(theta1-pi./2.0).*(3.7e+1./2.0e+2)+cos(theta2+pi./2.0).*(3.7e+1./2.0e+2)+3.0./2.5e+1).^2.*sign(cos(theta1-pi./2.0).*(3.7e+1./2.0e+2)+cos(theta2+pi./2.0).*(3.7e+1./2.0e+2)+3.0./2.5e+1).*sin(theta2+pi./2.0).*(sin(theta1-pi./2.0).*(3.7e+1./2.0e+2)+sin(theta2+pi./2.0).*(3.7e+1./2.0e+2)).*(3.7e+1./2.0e+2)))./((sin(theta1-pi./2.0).*(3.7e+1./2.0e+2)+sin(theta2+pi./2.0).*(3.7e+1./2.0e+2)).^2+abs(cos(theta1-pi./2.0).*(3.7e+1./2.0e+2)+cos(theta2+pi./2.0).*(3.7e+1./2.0e+2)+3.0./2.5e+1).^2)).*4.187654330625071e-1)./(cos(acos(sqrt((sin(theta1-pi./2.0).*(3.7e+1./2.0e+2)+sin(theta2+pi./2.0).*(3.7e+1./2.0e+2)).^2+abs(cos(theta1-pi./2.0).*(3.7e+1./2.0e+2)+cos(theta2+pi./2.0).*(3.7e+1./2.0e+2)+3.0./2.5e+1).^2).*(5.0e+1./3.7e+1))+atan2(sin(theta1-pi./2.0).*(-3.7e+1./2.0e+2)-sin(theta2+pi./2.0).*(3.7e+1./2.0e+2),abs(cos(theta1-pi./2.0).*(3.7e+1./2.0e+2)+cos(theta2+pi./2.0).*(3.7e+1./2.0e+2)+3.0./2.5e+1))+7.170057008954915e-2).*(-4.187654330625071e-1)+cos(theta2+pi./2.0).*(3.7e+1./2.0e+2)+3.0./5.0e+1)+(sin(theta2+pi./2.0).*(3.7e+1./2.0e+2)+sin(acos(sqrt((sin(theta1-pi./2.0).*(3.7e+1./2.0e+2)+sin(theta2+pi./2.0).*(3.7e+1./2.0e+2)).^2+abs(cos(theta1-pi./2.0).*(3.7e+1./2.0e+2)+cos(theta2+pi./2.0).*(3.7e+1./2.0e+2)+3.0./2.5e+1).^2).*(5.0e+1./3.7e+1))+atan2(sin(theta1-pi./2.0).*(-3.7e+1./2.0e+2)-sin(theta2+pi./2.0).*(3.7e+1./2.0e+2),abs(cos(theta1-pi./2.0).*(3.7e+1./2.0e+2)+cos(theta2+pi./2.0).*(3.7e+1./2.0e+2)+3.0./2.5e+1))+7.170057008954915e-2).*(1.0./sqrt((sin(theta1-pi./2.0).*(3.7e+1./2.0e+2)+sin(theta2+pi./2.0).*(3.7e+1./2.0e+2)).^2+abs(cos(theta1-pi./2.0).*(3.7e+1./2.0e+2)+cos(theta2+pi./2.0).*(3.7e+1./2.0e+2)+3.0./2.5e+1).^2).*(cos(theta2+pi./2.0).*(sin(theta1-pi./2.0).*(3.7e+1./2.0e+2)+sin(theta2+pi./2.0).*(3.7e+1./2.0e+2)).*(3.7e+1./1.0e+2)-abs(cos(theta1-pi./2.0).*(3.7e+1./2.0e+2)+cos(theta2+pi./2.0).*(3.7e+1./2.0e+2)+3.0./2.5e+1).*sign(cos(theta1-pi./2.0).*(3.7e+1./2.0e+2)+cos(theta2+pi./2.0).*(3.7e+1./2.0e+2)+3.0./2.5e+1).*sin(theta2+pi./2.0).*(3.7e+1./1.0e+2)).*1.0./sqrt((sin(theta1-pi./2.0).*(3.7e+1./2.0e+2)+sin(theta2+pi./2.0).*(3.7e+1./2.0e+2)).^2.*(-1.826150474799123)-abs(cos(theta1-pi./2.0).*(3.7e+1./2.0e+2)+cos(theta2+pi./2.0).*(3.7e+1./2.0e+2)+3.0./2.5e+1).^2.*1.826150474799123+1.0).*(2.5e+1./3.7e+1)+(abs(cos(theta1-pi./2.0).*(3.7e+1./2.0e+2)+cos(theta2+pi./2.0).*(3.7e+1./2.0e+2)+3.0./2.5e+1).^2.*((cos(theta2+pi./2.0).*(3.7e+1./2.0e+2))./abs(cos(theta1-pi./2.0).*(3.7e+1./2.0e+2)+cos(theta2+pi./2.0).*(3.7e+1./2.0e+2)+3.0./2.5e+1)+1.0./abs(cos(theta1-pi./2.0).*(3.7e+1./2.0e+2)+cos(theta2+pi./2.0).*(3.7e+1./2.0e+2)+3.0./2.5e+1).^2.*sign(cos(theta1-pi./2.0).*(3.7e+1./2.0e+2)+cos(theta2+pi./2.0).*(3.7e+1./2.0e+2)+3.0./2.5e+1).*sin(theta2+pi./2.0).*(sin(theta1-pi./2.0).*(3.7e+1./2.0e+2)+sin(theta2+pi./2.0).*(3.7e+1./2.0e+2)).*(3.7e+1./2.0e+2)))./((sin(theta1-pi./2.0).*(3.7e+1./2.0e+2)+sin(theta2+pi./2.0).*(3.7e+1./2.0e+2)).^2+abs(cos(theta1-pi./2.0).*(3.7e+1./2.0e+2)+cos(theta2+pi./2.0).*(3.7e+1./2.0e+2)+3.0./2.5e+1).^2)).*4.187654330625071e-1).*(sin(acos(sqrt((sin(theta1-pi./2.0).*(3.7e+1./2.0e+2)+sin(theta2+pi./2.0).*(3.7e+1./2.0e+2)).^2+abs(cos(theta1-pi./2.0).*(3.7e+1./2.0e+2)+cos(theta2+pi./2.0).*(3.7e+1./2.0e+2)+3.0./2.5e+1).^2).*(5.0e+1./3.7e+1))+atan2(sin(theta1-pi./2.0).*(-3.7e+1./2.0e+2)-sin(theta2+pi./2.0).*(3.7e+1./2.0e+2),abs(cos(theta1-pi./2.0).*(3.7e+1./2.0e+2)+cos(theta2+pi./2.0).*(3.7e+1./2.0e+2)+3.0./2.5e+1))+7.170057008954915e-2).*4.187654330625071e-1+sin(theta2+pi./2.0).*(3.7e+1./2.0e+2)).*1.0./(cos(acos(sqrt((sin(theta1-pi./2.0).*(3.7e+1./2.0e+2)+sin(theta2+pi./2.0).*(3.7e+1./2.0e+2)).^2+abs(cos(theta1-pi./2.0).*(3.7e+1./2.0e+2)+cos(theta2+pi./2.0).*(3.7e+1./2.0e+2)+3.0./2.5e+1).^2).*(5.0e+1./3.7e+1))+atan2(sin(theta1-pi./2.0).*(-3.7e+1./2.0e+2)-sin(theta2+pi./2.0).*(3.7e+1./2.0e+2),abs(cos(theta1-pi./2.0).*(3.7e+1./2.0e+2)+cos(theta2+pi./2.0).*(3.7e+1./2.0e+2)+3.0./2.5e+1))+7.170057008954915e-2).*(-4.187654330625071e-1)+cos(theta2+pi./2.0).*(3.7e+1./2.0e+2)+3.0./5.0e+1).^2).*(cos(acos(sqrt((sin(theta1-pi./2.0).*(3.7e+1./2.0e+2)+sin(theta2+pi./2.0).*(3.7e+1./2.0e+2)).^2+abs(cos(theta1-pi./2.0).*(3.7e+1./2.0e+2)+cos(theta2+pi./2.0).*(3.7e+1./2.0e+2)+3.0./2.5e+1).^2).*(5.0e+1./3.7e+1))+atan2(sin(theta1-pi./2.0).*(-3.7e+1./2.0e+2)-sin(theta2+pi./2.0).*(3.7e+1./2.0e+2),abs(cos(theta1-pi./2.0).*(3.7e+1./2.0e+2)+cos(theta2+pi./2.0).*(3.7e+1./2.0e+2)+3.0./2.5e+1))+7.170057008954915e-2).*(-4.187654330625071e-1)+cos(theta2+pi./2.0).*(3.7e+1./2.0e+2)+3.0./5.0e+1).^2)./((sin(acos(sqrt((sin(theta1-pi./2.0).*(3.7e+1./2.0e+2)+sin(theta2+pi./2.0).*(3.7e+1./2.0e+2)).^2+abs(cos(theta1-pi./2.0).*(3.7e+1./2.0e+2)+cos(theta2+pi./2.0).*(3.7e+1./2.0e+2)+3.0./2.5e+1).^2).*(5.0e+1./3.7e+1))+atan2(sin(theta1-pi./2.0).*(-3.7e+1./2.0e+2)-sin(theta2+pi./2.0).*(3.7e+1./2.0e+2),abs(cos(theta1-pi./2.0).*(3.7e+1./2.0e+2)+cos(theta2+pi./2.0).*(3.7e+1./2.0e+2)+3.0./2.5e+1))+7.170057008954915e-2).*4.187654330625071e-1+sin(theta2+pi./2.0).*(3.7e+1./2.0e+2)).^2+(cos(acos(sqrt((sin(theta1-pi./2.0).*(3.7e+1./2.0e+2)+sin(theta2+pi./2.0).*(3.7e+1./2.0e+2)).^2+abs(cos(theta1-pi./2.0).*(3.7e+1./2.0e+2)+cos(theta2+pi./2.0).*(3.7e+1./2.0e+2)+3.0./2.5e+1).^2).*(5.0e+1./3.7e+1))+atan2(sin(theta1-pi./2.0).*(-3.7e+1./2.0e+2)-sin(theta2+pi./2.0).*(3.7e+1./2.0e+2),abs(cos(theta1-pi./2.0).*(3.7e+1./2.0e+2)+cos(theta2+pi./2.0).*(3.7e+1./2.0e+2)+3.0./2.5e+1))+7.170057008954915e-2).*(-4.187654330625071e-1)+cos(theta2+pi./2.0).*(3.7e+1./2.0e+2)+3.0./5.0e+1).^2);
end

== matlab function MAIN_IC_TEST_original/MATLAB Function3 ==
  data: t input; theta1 input; turn_off output; theta2 input; knee_distance output
function [turn_off,knee_distance] = STOP(t,theta1,theta2)
    % End simulation if knees are too close 
    L1 = 18.5/100;
    L2 = 18.5/100;
    L5 = 12/100;
    q1 =  pi/2 - theta1; 
    q2 =  pi/2 - theta2;
    B1 = [-0.5*L5 - L1*cos(q1) ; L1*sin(q1)];
    B2 = [0.5*L5 + L2*cos(pi-q2) ; L2*sin(pi-q2)];
    knee_distance = abs(B1(1) - B2(1));
    if knee_distance<=0.10
        if t>=3.5
            turn_off = 1;
        else 
            turn_off = 0;
        end
    else 
        turn_off = 0;
    end

end

== matlab function MAIN_IC_TEST_original/MATLAB Function5 ==
  data: theta1 input; JT11 output; theta2 input; JT12 output; JT21 output; JT22 output
function [JT11,JT12,JT21,JT22] = Jacobian_Transpose(theta1,theta2)
%JACOBIAN_TRANSPOSE
%    [JT11,JT12,JT21,JT22] = JACOBIAN_TRANSPOSE(THETA1,THETA2)

%    This function was generated by the Symbolic Math Toolbox version 8.6.
%    13-May-2022 14:39:47

t2 = pi./2.0;
t3 = -t2;
t4 = t2+theta2;
t5 = t3+theta1;
t6 = cos(t4);
t7 = sin(t4);
t8 = cos(t5);
t9 = sin(t5);
t10 = t6.*(3.7e+1./2.0e+2);
t11 = t7.*(3.7e+1./2.0e+2);
t14 = t7.*1.85e-1i;
t12 = t8.*(3.7e+1./2.0e+2);
t13 = t9.*(3.7e+1./2.0e+2);
t15 = t9.*1.85e-1i;
t16 = -t14;
t17 = -t15;
t18 = t11+t13;
t20 = t10+t12+3.0./2.5e+1;
t19 = t18.^2;
t21 = abs(t20);
t22 = sign(t20);
t28 = t6.*t18.*(3.7e+1./1.0e+2);
t29 = t8.*t18.*(3.7e+1./1.0e+2);
t23 = t21.^2;
t24 = 1.0./t21;
t26 = t19.*1.826150474799123;
t35 = t16+t17+t21;
t42 = t7.*t21.*t22.*(3.7e+1./1.0e+2);
t43 = t9.*t21.*t22.*(3.7e+1./1.0e+2);
t25 = 1.0./t23;
t27 = -t26;
t30 = t23.*1.826150474799123;
t32 = t10.*t24;
t33 = t12.*t24;
t34 = t19+t23;
t36 = angle(t35);
t44 = -t42;
t45 = -t43;
t31 = -t30;
t37 = 1.0./t34;
t38 = sqrt(t34);
t48 = t11.*t18.*t22.*t25;
t49 = t13.*t18.*t22.*t25;
t50 = t28+t44;
t51 = t29+t45;
t39 = 1.0./t38;
t40 = t38.*(5.0e+1./3.7e+1);
t46 = t27+t31+1.0;
t52 = t32+t48;
t53 = t33+t49;
t41 = acos(t40);
t47 = 1.0./sqrt(t46);
t66 = t23.*t37.*t52;
t67 = t23.*t37.*t53;
t54 = t36+t41+7.170057008954915e-2;
t68 = t39.*t47.*t50.*(2.5e+1./3.7e+1);
t69 = t39.*t47.*t51.*(2.5e+1./3.7e+1);
t55 = cos(t54);
t56 = sin(t54);
t73 = t66+t68;
t74 = t67+t69;
t57 = t56.*4.187654330625071e-1;
t58 = t55.*4.187654330625071e-1;
t77 = t55.*t73.*(-4.187654330625071e-1);
t59 = -t58;
t60 = t11+t57;
t75 = t58.*t73;
t76 = t57.*t73;
t79 = t10+t77;
t61 = t60.^2;
t62 = t10+t59+3.0./5.0e+1;
t78 = t11+t76;
t63 = t62.^2;
t64 = 1.0./t62;
t65 = 1.0./t63;
t70 = t61+t63;
t71 = 1.0./t70;
t72 = 1.0./sqrt(t70);
JT11 = t72.*(t55.*t60.*t74.*8.375308661250142e-1+t56.*t62.*t74.*8.375308661250142e-1).*(-1.0./2.0);
if nargout > 1
    JT12 = t63.*t71.*(t58.*t64.*t74-t56.*t60.*t65.*t74.*4.187654330625071e-1);
end
if nargout > 2
    JT21 = (t72.*(t60.*t79.*2.0-t62.*t78.*2.0))./2.0;
end
if nargout > 3
    JT22 = -t63.*t71.*(t64.*t79+t60.*t65.*t78);
end

== matlab function MAIN_IC_TEST_original/MATLAB Function6 ==
  data: E output; r input; phi input; r_ref input; phi_ref input; dE output; dr input; dphi input
function [E,dE] = Error(r,phi,r_ref,phi_ref,dr,dphi)
    
    dr_ref = 0.0;
    dphi_ref = 0.0;
    
    E = [r_ref - r; phi_ref - phi];
    dE = [dr_ref - dr; dphi_ref - dphi];
    
end

== matlab function MAIN_IC_TEST_original/MATLAB Function7 ==
  data: w output; E input; dE input
function w  = Controller(E,dE)
    Kp_r = 200;  
    Kp_phi = 0;  
    Kd_r = 0.1;  
    Kd_phi = 0.0;

    wr = Kp_r*E(1) + Kd_r*dE(1);
    wphi = Kp_phi*E(2) + Kd_phi*dE(2);
    
    w = [wr;wphi];
end

== matlab function MAIN_IC_TEST_original/MATLAB Function8 ==
  data: tau1 output; w input; JT11 input; tau2 output; JT12 input; JT21 input; JT22 input
function [tau1,tau2]  = Mapping(w,JT11,JT12,JT21,JT22)
    JT = [JT11,JT12;JT21,JT22];
    tau = JT*w;
    tau1 = tau(1);
    tau2 = tau(2);
end

== matlab function MAIN_IC_TEST_original/to_Polar1 ==
  data: theta1 input; theta2 input; r output; phi output
function [r,phi] = Position(theta1,theta2)
%POSITION
%    [R,PHI] = POSITION(THETA1,THETA2)

%    This function was generated by the Symbolic Math Toolbox version 8.6.
%    13-May-2022 14:39:46

r = sqrt((sin(acos(sqrt((sin(theta1-pi./2.0).*(3.7e+1./2.0e+2)+sin(theta2+pi./2.0).*(3.7e+1./2.0e+2)).^2+abs(cos(theta1-pi./2.0).*(3.7e+1./2.0e+2)+cos(theta2+pi./2.0).*(3.7e+1./2.0e+2)+3.0./2.5e+1).^2).*(5.0e+1./3.7e+1))+atan2(sin(theta1-pi./2.0).*(-3.7e+1./2.0e+2)-sin(theta2+pi./2.0).*(3.7e+1./2.0e+2),abs(cos(theta1-pi./2.0).*(3.7e+1./2.0e+2)+cos(theta2+pi./2.0).*(3.7e+1./2.0e+2)+3.0./2.5e+1))+7.170057008954915e-2).*4.187654330625071e-1+sin(theta2+pi./2.0).*(3.7e+1./2.0e+2)).^2+(cos(acos(sqrt((sin(theta1-pi./2.0).*(3.7e+1./2.0e+2)+sin(theta2+pi./2.0).*(3.7e+1./2.0e+2)).^2+abs(cos(theta1-pi./2.0).*(3.7e+1./2.0e+2)+cos(theta2+pi./2.0).*(3.7e+1./2.0e+2)+3.0./2.5e+1).^2).*(5.0e+1./3.7e+1))+atan2(sin(theta1-pi./2.0).*(-3.7e+1./2.0e+2)-sin(theta2+pi./2.0).*(3.7e+1./2.0e+2),abs(cos(theta1-pi./2.0).*(3.7e+1./2.0e+2)+cos(theta2+pi./2.0).*(3.7e+1./2.0e+2)+3.0./2.5e+1))+7.170057008954915e-2).*(-4.187654330625071e-1)+cos(theta2+pi./2.0).*(3.7e+1./2.0e+2)+3.0./5.0e+1).^2);
if nargout > 1
    phi = pi./2.0-angle(cos(acos(sqrt((sin(theta1-pi./2.0).*(3.7e+1./2.0e+2)+sin(theta2+pi./2.0).*(3.7e+1./2.0e+2)).^2+abs(cos(theta1-pi./2.0).*(3.7e+1./2.0e+2)+cos(theta2+pi./2.0).*(3.7e+1./2.0e+2)+3.0./2.5e+1).^2).*(5.0e+1./3.7e+1))+atan2(sin(theta1-pi./2.0).*(-3.7e+1./2.0e+2)-sin(theta2+pi./2.0).*(3.7e+1./2.0e+2),abs(cos(theta1-pi./2.0).*(3.7e+1./2.0e+2)+cos(theta2+pi./2.0).*(3.7e+1./2.0e+2)+3.0./2.5e+1))+7.170057008954915e-2).*(-4.187654330625071e-1)+sin(acos(sqrt((sin(theta1-pi./2.0).*(3.7e+1./2.0e+2)+sin(theta2+pi./2.0).*(3.7e+1./2.0e+2)).^2+abs(cos(theta1-pi./2.0).*(3.7e+1./2.0e+2)+cos(theta2+pi./2.0).*(3.7e+1./2.0e+2)+3.0./2.5e+1).^2).*(5.0e+1./3.7e+1))+atan2(sin(theta1-pi./2.0).*(-3.7e+1./2.0e+2)-sin(theta2+pi./2.0).*(3.7e+1./2.0e+2),abs(cos(theta1-pi./2.0).*(3.7e+1./2.0e+2)+cos(theta2+pi./2.0).*(3.7e+1./2.0e+2)+3.0./2.5e+1))+7.170057008954915e-2).*4.187654330625071e-1i+cos(theta2+pi./2.0).*(3.7e+1./2.0e+2)+sin(theta2+pi./2.0).*1.85e-1i+3.0./5.0e+1);
end

== matlab function MAIN_IC_TEST_original/Subsystem1/Motor 3 Write - THETA1/MATLAB Function ==
  data: p_des input; P8H output; v_des input; kp input; kd input; t_ff input; P8L output; V8H output; V4L output; KP4H output; KP8L output; KD8H output; KD4L output; T4H output; T8L output
function [P8H,P8L,V8H,V4L,KP4H,KP8L,KD8H,KD4L,T4H,T8L] = AK1090(p_des, v_des, kp, kd, t_ff)
    % Coppied from AK70-10 manual
    % NB: CONSTANTS FOR AK70-10
    p_min = -12.5; % rad
    p_max = +12.5; % rad
    v_min = -50.0; % rad/s
    v_max = +50.0; % rad/s
    t_min = -65.0; % Nm
    t_max = +65.0; % Nm
    kp_min = 0;
    kp_max = 500;
    kd_min = 0;
    kd_max = 5;
    
    % bound inputs
    p_des = min([max([p_min,p_des]),p_max]);
    v_des = min([max([v_min,v_des]),v_max]);
    kp = min([max([kp_min,kp]),kp_max]);
    kd = min([max([kd_min,kd]),kd_max]);
    t_ff = min([max([t_min,t_ff]),t_max]);
    
    % convert floats to unsigned integers
    p_int = float_to_uint(p_des, p_min, p_max, 16);
    v_int = float_to_uint(v_des, v_min, v_max, 12);
    kp_int = float_to_uint(kp, kp_min, kp_max, 12);
    kd_int = float_to_uint(kd, kd_min, kd_max, 12);
    t_int = float_to_uint(t_ff, t_min, t_max, 12);
    
    % break up for CAN frame 
    P8H = bitshift(p_int, -8); % 8 higher bits
    P8L = bitand(p_int, 0xFF); % 8 lower bits
    V8H = bitshift(v_int, -4); % 8 higher bits
    V4L = bitand(v_int, 0xF); % 4 lower bits
    KP4H = bitshift(kp_int, -8); % 4 higher bits
    KP8L = bitand(kp_int, 0xFF); % 8 lower bits
    KD8H = bitshift(kd_int, -4); % 8 higher bits
    KD4L = bitand(kd_int, 0xF); % 4 lower bits
    T4H = bitshift(t_int, -8); % 4 higher bits
    T8L = bitand(t_int, 0xFF); % 8 lower bits
    
    % Converts a float to an unsigned int, given range and number of bits
    function x_int = float_to_uint(x, x_min, x_max, n_bits)
        span = x_max - x_min;
        min([max([x_min,x]),x_max])
        x_int = ((x - x_min)*(bitshift(1, n_bits) / span));
    end
end
%final_values = desired_pos,desired_vel,desired_kp,desired_kd,desired_tau;
